simulink model "tp1_simulink_e_g"  (R2024a)
settings: Solver=VariableStepAuto  StartTime=0.0  StopTime=10.0  RelTol=1e-3
values from neighbouring files (symbols this model uses):
  x0 = [1; 0; m*g]    [tp1_v2.m]
libraries: cstblocks x1
settings Model: Creator=tiago  LastModifiedBy=tiago

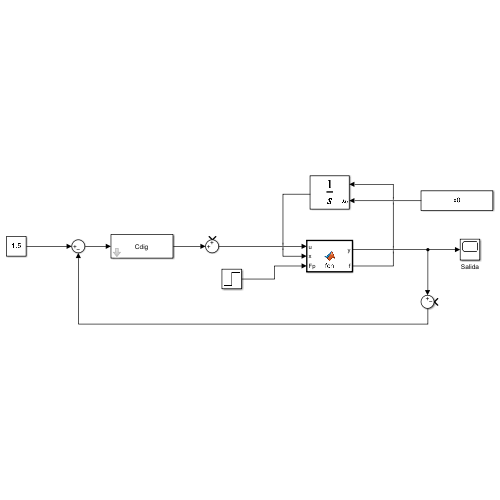
[thumbnail: Simulink's stored preview of the top-level diagram]
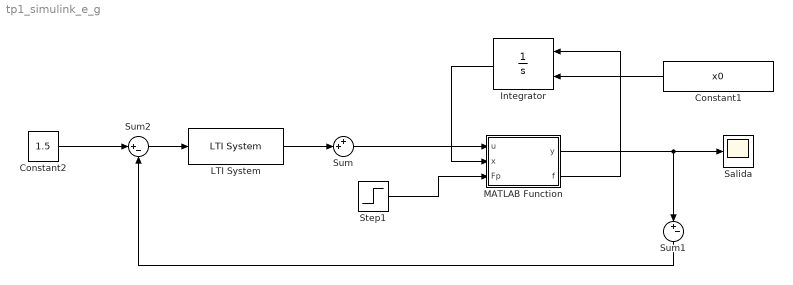
== system tp1_simulink_e_g ==
  Constant1 : Constant  Value=x0
  Constant2 : Constant  Value=1.5
  Integrator : Integrator  InitialConditionSource=external
  LTI System : cstblocks/LTI System  sys=Cdig  IC=[]  PadeOrder=0
  MATLAB Function : MATLAB Function  TreatAsAtomicUnit=on
  Salida : Scope
  Step1 : Step  After=0.5  SampleTime=0
  Sum : Sum  Inputs=++|
  Sum1 : Sum  Inputs=|+-
  Sum2 : Sum  Inputs=|+-
  wires:
  Sum2/1 -> LTI System/1
  Sum1/1 -> Sum2/2
  Constant2/1 -> Sum2/1
  Step1/1 -> MATLAB Function/3(Fp)
  Sum/1 -> MATLAB Function/1(u)
  Constant1/1 -> Integrator/2
  LTI System/1 -> Sum/2
  MATLAB Function/2(f) -> Integrator/1
  Integrator/1 -> MATLAB Function/2(x)
  MATLAB Function/1(y) -> Sum1/1, Salida/1

== matlab function tp1_simulink_e_g/MATLAB Function ==
  data: u input; y output; x input; f output; Fp input
function [y,f] = fcn(u, x, Fp)
    %Constantes
    m = 0.1;
    R = 4;
    g = 10;
    L = 0.01;
    
    %Ecuaciones no lineales
    F1 = x(2);
    F2 = g - x(3) / (m * x(1));
    F3 = u/L - R * x(3)/L;

    y = x(1);
    f = [F1 F2 F3];
